simulink model "A10_28"  (R2024b)
settings: Solver=VariableStepAuto  StartTime=0.0  StopTime=500  MaxStep=0.001  RelTol=1e-3
settings Model: Creator=Administrator  LastModifiedBy=Administrator

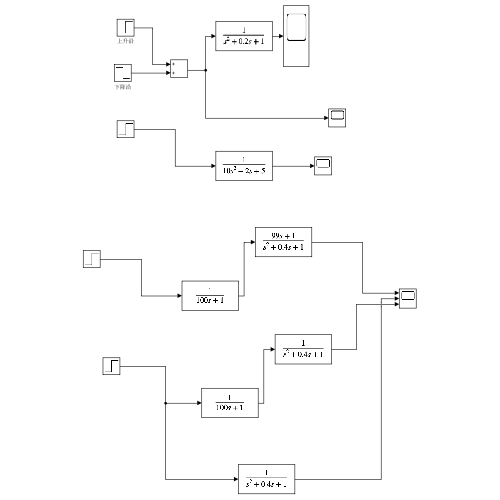
[thumbnail: Simulink's stored preview of the top-level diagram]
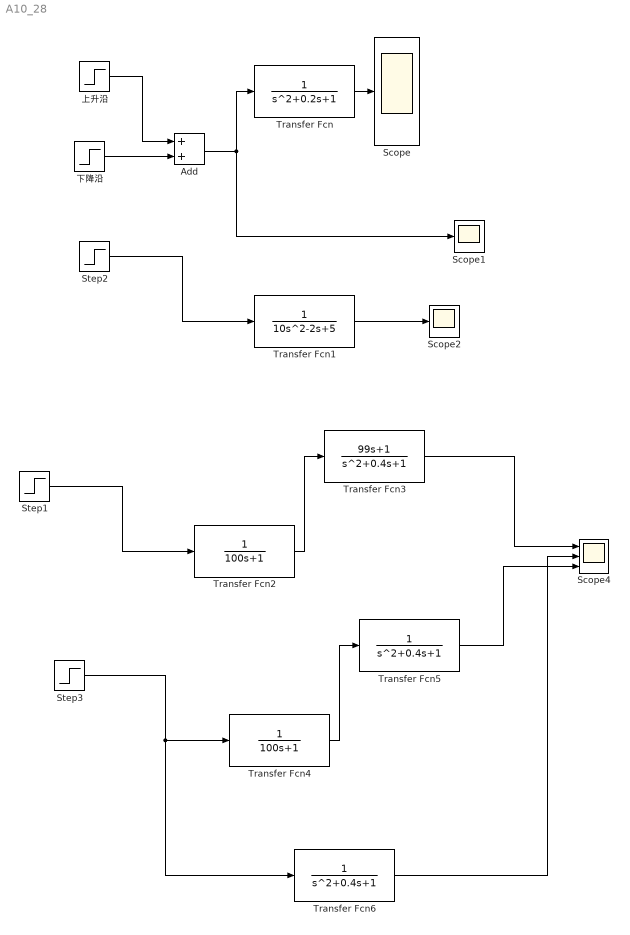
== system A10_28 ==
  Add : Sum
  Scope : Scope
  Scope1 : Scope
  Scope2 : Scope
  Scope4 : Scope  NumInputPorts=3
  Step1 : Step  After=500  SampleTime=0
  Step2 : Step  After=0.000000000000000000000000000000000000000000000000000000000000000000000000000000000000000000000001  SampleTime=0
  Step3 : Step  After=500  SampleTime=0
  Transfer Fcn : TransferFcn  Denominator=[1 0.2 1]
  Transfer Fcn1 : TransferFcn  Denominator=[10 -2 5]
  Transfer Fcn2 : TransferFcn  Denominator=[100,1]
  Transfer Fcn3 : TransferFcn  Numerator=[99 1]  Denominator=[1 0.4 1]
  Transfer Fcn4 : TransferFcn  Denominator=[100,1]
  Transfer Fcn5 : TransferFcn  Denominator=[1 0.4 1]
  Transfer Fcn6 : TransferFcn  Denominator=[1 0.4 1]
  上升沿 : Step  Time=5  After=10  SampleTime=0
  下降沿 : Step  Time=5.1  After=-10  SampleTime=0
  wires:
  上升沿/1 -> Add/1
  下降沿/1 -> Add/2
  Add/1 -> Scope1/1, Transfer Fcn/1
  Transfer Fcn/1 -> Scope/1
  Transfer Fcn1/1 -> Scope2/1
  Step2/1 -> Transfer Fcn1/1
  Transfer Fcn2/1 -> Transfer Fcn3/1
  Step1/1 -> Transfer Fcn2/1
  Transfer Fcn3/1 -> Scope4/1
  Transfer Fcn4/1 -> Transfer Fcn5/1
  Transfer Fcn5/1 -> Scope4/3
  Step3/1 -> Transfer Fcn6/1, Transfer Fcn4/1
  Transfer Fcn6/1 -> Scope4/2
